simulink model "test_1"  (R2022a)
settings: Solver=ode4  StartTime=0.0  StopTime=50  FixedStep=0.01  RelTol=1e-3
libraries: simulink x1
settings Model: Creator=Alireza Sharifi  LastModifiedBy=Alireza Sharifi

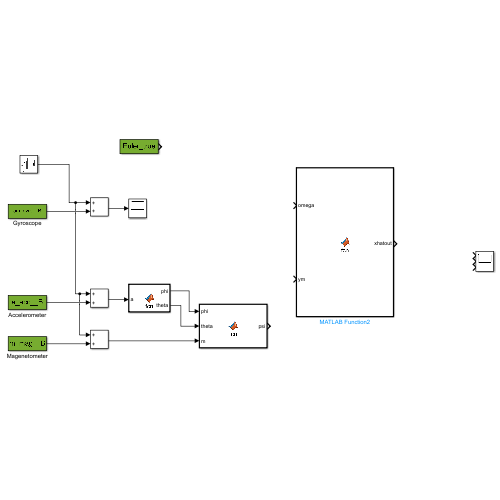
[thumbnail: Simulink's stored preview of the top-level diagram]
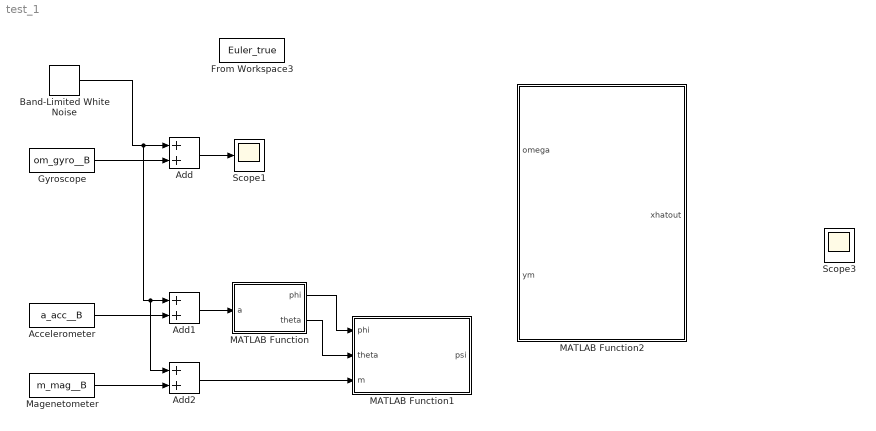
== system test_1 ==
  Accelerometer : FromWorkspace  VariableName=a_acc__B  SampleTime=0.01
  Add : Sum
  Add1 : Sum
  Add2 : Sum
  Band-Limited White Noise : simulink/Sources/Band-Limited White Noise  Cov=1e-5  Ts=0.01  seed=[23341]
  From Workspace3 : FromWorkspace  VariableName=Euler_true  SampleTime=0.01
  Gyroscope : FromWorkspace  VariableName=om_gyro__B  SampleTime=0.01
  MATLAB Function : MATLAB Function  TreatAsAtomicUnit=on
  MATLAB Function1 : MATLAB Function  TreatAsAtomicUnit=on
  MATLAB Function2 : MATLAB Function  TreatAsAtomicUnit=on
  Magenetometer : FromWorkspace  VariableName=m_mag__B  SampleTime=0.01
  Scope1 : Scope
  Scope3 : Scope  NumInputPorts=3
  wires:
  Gyroscope/1 -> Add/2
  Add/1 -> Scope1/1
  Accelerometer/1 -> Add1/2
  Magenetometer/1 -> Add2/2
  Band-Limited White Noise/1 -> Add2/1, Add1/1, Add/1
  Add1/1 -> MATLAB Function/1(a)
  Add2/1 -> MATLAB Function1/3(m)
  MATLAB Function/2(theta) -> MATLAB Function1/2(theta)
  MATLAB Function/1(phi) -> MATLAB Function1/1(phi)

== matlab function test_1/MATLAB Function1 ==
  data: phi input; psi output; theta input; m input
function psi = fcn(phi,theta,m)
mx=m(1);
my=m(2);
mz=m(3);
%
num_psi=-cos(phi)*my+sin(phi)*mz;
den_psi=cos(theta)*mx+sin(theta)*sin(phi)*my+sin(theta)*cos(phi)*mz;
declination_angle=-4.0266*pi/180;
psi=atan2(num_psi,den_psi)+declination_angle;

== matlab function test_1/MATLAB Function ==
  data: a input; phi output; theta output
function [phi,theta] = fcn(a)
ax=a(1);
ay=a(2);
az=a(3);
g=9.81;
phi=atan2(-ay,-az);
theta=asin(ax/g);

== matlab function test_1/MATLAB Function2 ==
  data: omega input; xhatout output; ym input
function xhatout = fcn(omega,ym)
p=omega(1);
q=omega(2);
r=omega(3);
%%
persistent xhat P
if isempty(xhat)
    xhat=[0;0;0];
end
if isempty(P)
    P=[100 0 0;
        0  100 0;
        0  0   100];
end
%%
Ts=0.01;
Q=[1 0 0;
        0  1 0;
        0  0   1];
R=0.01*[1 0 0;
        0  1 0;
        0  0   1];
%%
xhat1=xhat(1)+Ts*(p+tan(xhat(2))*sin(xhat(1))*q+r*cos(xhat(1))*tan(xhat(2)));
xhat2=xhat(2)+Ts*(q*cos(xhat(1))-r*sin(xhat(1)));
xhat3=xhat(3)+Ts*(sec(xhat(2))*(q*sin(xhat(1))+r*cos(xhat(1))));
%%
xhat=[xhat1;xhat2;xhat3];
%%
F=[1+Ts*tan(xhat(2))*(q*cos(xhat(1))-r*sin(xhat(1))) ...
    Ts*(q*sin(xhat(1))+r*cos(xhat(1)))/(cos(xhat(2))^2) 0;
  Ts*(-q*sin(xhat(1))-r*cos(xhat(1)))   1   0;
  Ts*(q*cos(xhat(1))-r*sin(xhat(1)))/cos(xhat(2)) ...
     Ts*sin(xhat(2))*(q*sin(xhat(1))+r*cos(xhat(1)))/(cos(xhat(2))^2) 1];
Gama=[Ts Ts*tan(xhat(2))*sin(xhat(1)) Ts*tan(xhat(2))*cos(xhat(1));
    0  Ts*cos(xhat(1))  -Ts*sin(xhat(1));
    0  Ts*sin(xhat(1))/cos(xhat(2)) Ts*cos(xhat(1))/cos(xhat(2))];
P=F*P*F'+Gama*Q*Gama';
%%
C=[1 0 0;
    0 1 0;
    0 0 1];
yhat=C*xhat;
K=P*C'*inv(C*P*C'+R);
xhat=xhat+K(ym-yhat);
P=(eye(3)-K*C)*P*(eye(3)-K*C)'+K*R*K';
xhatout=xhat;
